simulink model "zad73_kaskadaslx"  (R2015a)
settings: Solver=FixedStepDiscrete  StartTime=0.0  StopTime=99.0  FixedStep=1  RelTol=1e-3
settings Model: Creator=Bojana Vasic  LastModifiedBy=Bojana Vasic

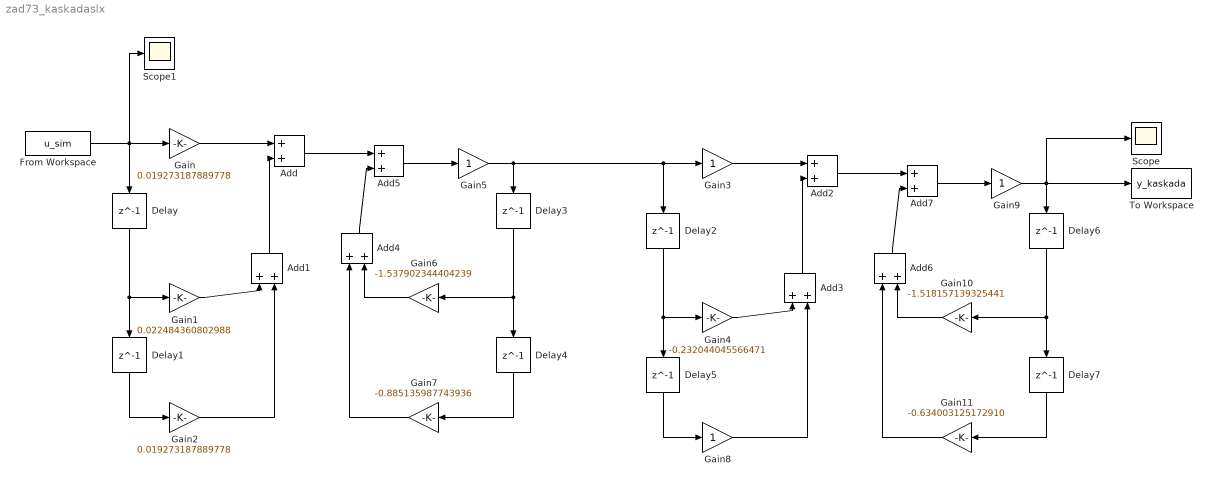
== system zad73_kaskadaslx ==
  Add{,1..7} (8 alike) : Sum
  Delay{,1..7} (8 alike) : Delay  DelayLength=1
  From Workspace : FromWorkspace  VariableName=u_sim  SampleTime=1
  Gain : Gain  Gain=0.019273187889778
  Gain1 : Gain  Gain=0.022484360802988
  Gain10 : Gain  Gain=-1.518157139325441
  Gain11 : Gain  Gain=-0.634003125172910
  Gain2 : Gain  Gain=0.019273187889778
  Gain{3,5,8..9} (4 alike) : Gain
  Gain4 : Gain  Gain=-0.232044045566471
  Gain6 : Gain  Gain=-1.537902344404239
  Gain7 : Gain  Gain=-0.885135987743936
  Scope : Scope
  Scope1 : Scope
  To Workspace : ToWorkspace  VariableName=y_kaskada  SampleTime=-1
      settings: Save2DSignal=2-D array (concatenate along first dimension)
  wires:
  Gain/1 -> Add/1
  Add/1 -> Add5/1
  Add4/1 -> Add5/2
  Gain6/1 -> Add4/2
  Delay3/1 -> Delay4/1, Gain6/1
  Add5/1 -> Gain5/1
  Delay4/1 -> Gain7/1
  From Workspace/1 -> Delay/1, Scope1/1, Gain/1
  Delay/1 -> Delay1/1, Gain1/1
  Delay1/1 -> Gain2/1
  Gain1/1 -> Add1/1
  Add1/1 -> Add/2
  ? -> ?
  Gain2/1 -> Add1/2
  Gain7/1 -> Add4/1
  Gain3/1 -> Add2/1
  Add2/1 -> Add7/1
  Add6/1 -> Add7/2
  Gain10/1 -> Add6/2
  Delay6/1 -> Delay7/1, Gain10/1
  Add7/1 -> Gain9/1
  Delay7/1 -> Gain11/1
  Gain5/1 -> Delay2/1, Gain3/1, Delay3/1
  Delay2/1 -> Delay5/1, Gain4/1
  Delay5/1 -> Gain8/1
  Gain4/1 -> Add3/1
  Add3/1 -> Add2/2
  Gain8/1 -> Add3/2
  Gain11/1 -> Add6/1
  Gain9/1 -> Scope/1, To Workspace/1, Delay6/1
